simulink model "TMP_MPC_Arduino"  (R2025b)
settings: Solver=FixedStepAuto  StartTime=0.0  StopTime=10.0  RelTol=1e-3
libraries: arduinolib x2, mpclib x1, slctrl_signal x1
settings Model: ExtModeTrigDuration=2  Creator=geokr  LastModifiedBy=geokr
settings SolverCC: AutoInsertRateTranBlk=on
settings OptimizationCC: EnhancedBackFolding=on  PassReuseOutputArgsAs=Individual arguments  ZeroExternalMemoryAtStartup=off  ZeroInternalMemoryAtStartup=off  MaxStackSize=64  OptimizeBlockOrder=speed  DifferentSizesBufferReuse=on  OptimizationCustomize=off  EfficientTunableParamExpr=on
settings DebuggingCC: ParameterTunabilityLossMsg=error
settings HardwareCC: ProdBitPerInt=16.0  ProdBitPerPointer=16.0  ProdBitPerSizeT=16.0  ProdBitPerPtrDiffT=16.0  ProdLargestAtomicFloat=None  ProdWordSize=8.0  ProdHWDeviceType=Atmel->AVR
settings SFSimCC: MATLABDynamicMemAlloc=off
settings RTWCC: SystemTargetFile=ert.tlc  HardwareBoard=Arduino Uno  TemplateMakefile=ert_default_tmf  Toolchain=Arduino AVR  Description=Embedded Coder
settings CodeAppCC: ForceParamTrailComments=on  IgnoreCustomStorageClasses=off  OperatorAnnotations=on  SimulinkDataObjDesc=on  SFDataObjDesc=on  InsertBlockDesc=on
settings ERTTargetCC: ExtModeTransport=3.0  ExtModeStaticAlloc=on  ExtModeAutomaticAllocSize=off  ExtModeStaticAllocSize=250.0  ExtModeMexFile=ext_xcp  ExtModeIntrfLevel=Level2 - Open  InlinedParameterPlacement=Hierarchical  SupportContinuousTime=on  SupportVariableSizeSignals=on

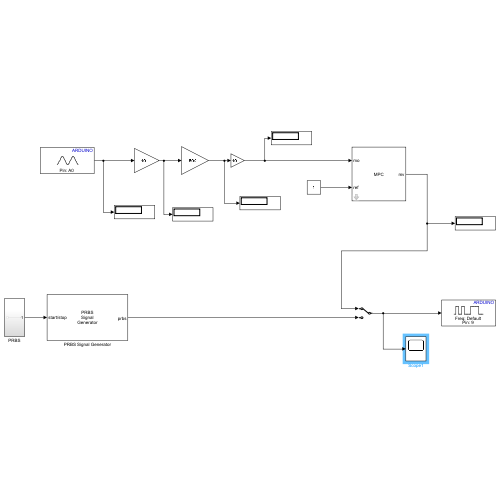
[thumbnail: Simulink's stored preview of the top-level diagram]
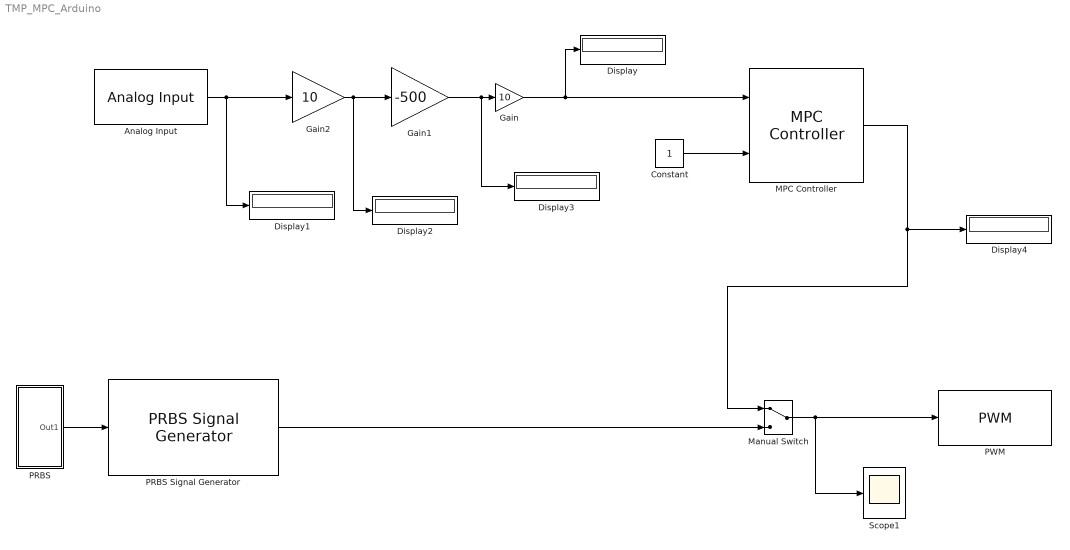
== system TMP_MPC_Arduino ==
  Analog Input : arduinolib/Analog Input  pinNumber=0  ReadResultsOnly=off  ConversionTriggerSource=Software  ExternalTriggerType=uint32( 0 )  OutputDataType=uint16  EnableConversionCompleteNotify=off  EnableOuputStatus=off  SampleTime=-1  blockPlatform=arduino
      settings: LibrarySourceBlock=gizmoLibrary/Arduino Utilities/Analog Input
  Constant : Constant
  Display{,1..4} (5 alike) : Display
  Gain : Gain  Gain=10
  Gain1 : Gain  Gain=-500
  Gain2 : Gain  Gain=10
  MPC Controller : mpclib/MPC Controller  SCDEnableBlockLinearizationSpecification=on  is_multiple=0  enable_value=0  return_u0=off  updateMPCinCallerWorkspace=on  md_inport=off  mv_inport=off  uref_inport=off  return_cost=off  return_mvseq=off  return_qpstatus=off  return_xseq=off  return_state=off  return_ovseq=off  state_inport=off  umin_inport=off  umax_inport=off  ymin_inport=off  ymax_inport=off  cc_inport=off  ywt_inport=off  uwt_inport=off  duwt_inport=off  rhoeps_inport=off  pm_inport=off  MaximumP=10  HorizonChoice=FixedHorizon  n_ts=1  n_p=10  n_mv=1  n_md=1  n_ud=0  n_mo=1  n_uo=0  BlockDataType=double  SampleTimeInherited=off  switch_inport=off
  Manual Switch : ManualSwitch
  PRBS : Subsystem
  PRBS Signal Generator : slctrl_signal/PRBS Signal Generator  DiscreteTs=0.1  BlockDataType=double  SignalSource=Block parameters  Frequencies=[0.5 1 2]  FreqUnits=rad/s  Amplitudes=1  NumOfFreq=3  NumOfPRBSPeriod=1  UseAutogenNumOfPRBSPeriod=off  PRBSSignalOrder=12  UseAutogenPRBSSignalOrder=off  UseExternalTs=off  CompiledTsChoice=InternalTs
      settings: LibrarySourceBlock=slctrlblks/Signal Generation/PRBS Signal Generator
  PWM : arduinolib/PWM  pinNumber=9  frequencyType=Default  desiredFrequency=50  achievableFrequency=490.2
      settings: LibrarySourceBlock=gizmoLibrary/Arduino Utilities/PWM
  Scope1 : Scope
  wires:
  Constant/1 -> MPC Controller/2
  Manual Switch/1 -> Scope1/1, PWM/1
  MPC Controller/1 -> Manual Switch/1, Display4/1
  PRBS Signal Generator/1 -> Manual Switch/2
  Gain1/1 -> Display3/1, Gain/1
  Gain/1 -> Display/1, MPC Controller/1
  Gain2/1 -> Display2/1, Gain1/1
  Analog Input/1 -> Display1/1, Gain2/1
  PRBS/1(Out1) -> PRBS Signal Generator/1

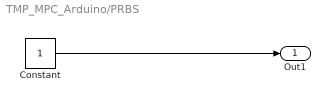
== system TMP_MPC_Arduino/PRBS ==
  Constant : Constant
  Out1 : Outport
  wires:
  Constant/1 -> Out1/1
